simulink model "problem1"  (R2020a)
settings: Solver=VariableStepAuto  StartTime=0.0  StopTime=200  RelTol=1e-3
libraries: simulink x1
settings Model: Creator=Jake  LastModifiedBy=Jake

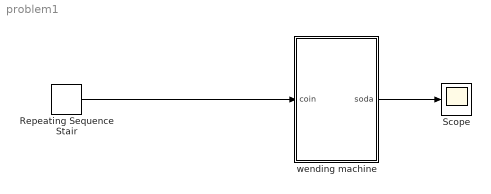
== system problem1 ==
  Repeating Sequence Stair : simulink/Sources/Repeating Sequence Stair  OutValues=[3 1 4 2 1].'  tsamp=-1  OutMin=[]  OutMax=[]  OutDataTypeStr=double  OutputDataTypeScalingMode=double  OutDataType=fixdt(0,8)  ConRadixGroup=Best Precision: Vector-wise  OutScaling=2^-12
  Scope : Scope
  wending machine : Stateflow chart  TreatAsAtomicUnit=on
  wires:
  wending machine/1(soda) -> Scope/1
  Repeating Sequence Stair/1 -> wending machine/1(coin)

== stateflow chart problem1/wending machine ==
  state nothing
  state nickel
  state dime
  (default) -> nothing
  nothing -> nickel [order 1] : [coin==1]{soda=0}
  nickel -> nothing [order 1] : [coin==2]{soda=1}
  dime -> nothing [order 1] : [coin==1]{soda=1}
  nothing -> dime [order 2] : [coin==2]{soda=0}
  nickel -> dime [order 2] : [coin==1]{soda==0}
  dime -> nickel [order 2] : [coin==2]{soda=1}
  data: coin input; soda output
